simulink model "ModeloSistema"  (R2012b)
settings: Solver=ode3  StartTime=0.0  StopTime=100  FixedStep=1e-4  RelTol=1e-3
undefined symbols (not defined in the file or in its folder): Control_02_Discreto_zpk, Planta_sistema_3
settings Model: Creator=Augusto  LastModifiedBy=Augusto

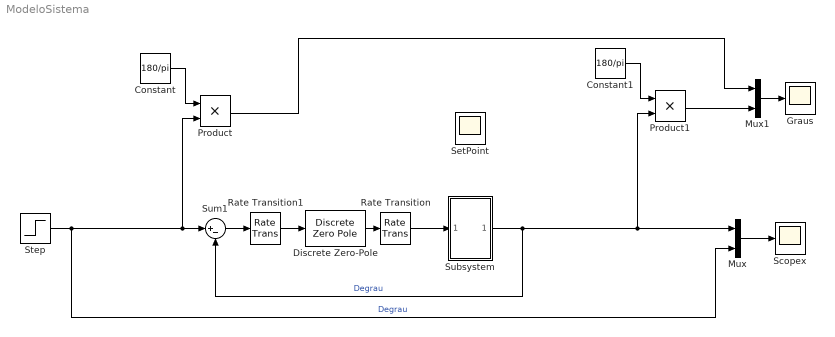
== system ModeloSistema ==
  Constant : Constant  Value=180/pi
  Constant1 : Constant  Value=180/pi
  Discrete Zero-Pole : DiscreteZeroPole  Zeros=Control_02_Discreto_zpk.z{1}  Poles=Control_02_Discreto_zpk.p{1}  Gain=Control_02_Discreto_zpk.k  SampleTime=0.2
  Graus : Scope
      settings: TimeRange=100  YMin=-0  YMax=120  SaveName=ScopeData3
  Mux : Mux  Inputs=2
  Mux1 : Mux  Inputs=2
  Product : Product  RndMeth=Zero
  Product1 : Product  RndMeth=Zero
  Rate Transition : RateTransition
  Rate Transition1 : RateTransition  OutPortSampleTime=0.2
  Scopex : Scope
      settings: TimeRange=30  YMin=-5250  YMax=250  SaveName=ScopeData5
  SetPoint : Scope
      settings: TimeRange=150  YMin=14  YMax=30
  Step : Step  Time=0  After=pi/2  SampleTime=0
  Subsystem : Subsystem
  Sum1 : Sum  Inputs=|+-
  wires:
  Step/1 -> Product/2, Sum1/1, Mux/2  "Degrau"
  Mux/1 -> Scopex/1
  Constant/1 -> Product/1
  Subsystem/1(Out1) -> Product1/2, Mux/1, Sum1/2  "Degrau"
  Constant1/1 -> Product1/1
  Product1/1 -> Mux1/2
  Product/1 -> Mux1/1
  Mux1/1 -> Graus/1
  Discrete Zero-Pole/1 -> Rate Transition/1
  Rate Transition1/1 -> Discrete Zero-Pole/1
  Rate Transition/1 -> Subsystem/1(In1)
  Sum1/1 -> Rate Transition1/1

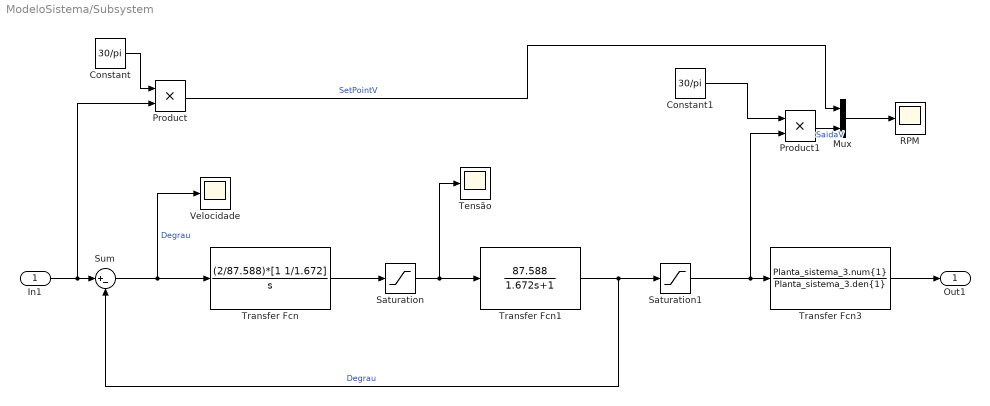
== system ModeloSistema/Subsystem ==
  In1 : Inport
  Constant : Constant  Value=30/pi
  Constant1 : Constant  Value=30/pi
  Mux : Mux  Inputs=2
  Product : Product  RndMeth=Zero
  Product1 : Product  RndMeth=Zero
  RPM : Scope
      settings: ShowLegends=on  TimeRange=50  YMin=-1000  YMax=4000  SaveName=ScopeData6
  Saturation : Saturate  UpperLimit=11.4  LowerLimit=-11.4
  Saturation1 : Saturate  UpperLimit=10000*pi/30  LowerLimit=-10000*pi/30
  Sum : Sum  Inputs=|+-
  Tensão : Scope
      settings: TimeRange=30  YMin=-4  YMax=12  SaveName=ScopeData4
  Transfer Fcn : TransferFcn  Numerator=(2/87.588)*[1 1/1.672]  Denominator=[1 0]
  Transfer Fcn1 : TransferFcn  Numerator=[87.588]  Denominator=[1.672 1]
  Transfer Fcn3 : TransferFcn  Numerator=Planta_sistema_3.num{1}  Denominator=Planta_sistema_3.den{1}
  Velocidade : Scope
  Out1 : Outport
  wires:
  In1/1 -> Product/2, Sum/1
  Transfer Fcn/1 -> Saturation/1
  Saturation/1 -> Tensão/1, Transfer Fcn1/1
  Transfer Fcn3/1 -> Out1/1
  Sum/1 -> Velocidade/1, Transfer Fcn/1  "Degrau"
  Constant/1 -> Product/1
  Transfer Fcn1/1 -> Sum/2, Saturation1/1  "Degrau"
  Constant1/1 -> Product1/1
  Product1/1 -> Mux/2  "SaidaV"
  Mux/1 -> RPM/1
  Product/1 -> Mux/1  "SetPointV"
  Saturation1/1 -> Transfer Fcn3/1, Product1/2
